simulink model "swcBrakePedalSignalingApp"  (R2022b)
settings: Solver=FixedStepDiscrete  StartTime=0  StopTime=10.0  FixedStep=0.01  RelTol=1e-3
values from neighbouring files (symbols this model uses):
  C_stopLightsSpeedThresholdSafety = Simulink.Parameter    [swcBrakePedalSignalingApp_defineIntCalibs.m]    (also in swcStopLightsMgr_defineIntCalibs.m)
  usageId = Simulink.Signal    [swcStopLightsMgr_defineIntCalibs.m]
undefined symbols (not defined in the file or in its folder): Init_stopLightASILB, pattern, STEP_BrakePedalSignalingApp, STOPLIGHTS_USAGES_DRIVER_BRAKE_PEDAL, STOPLIGHTS_USAGES_ESP_REQUEST, STOPLIGHTS_USAGES_PDC_REQUEST, usageAction, valueState
libraries: Ampere_Library x12, simulink x1
settings Model: ModifiedByFormat=Smrithi Pai  Creator=Smrithi Pai  LastModifiedBy=Smrithi Pai
settings DataIOCC: SaveOutput=off  SignalLogging=off  DSMLogging=off  SaveTime=off  ReturnWorkspaceOutputs=off
settings OptimizationCC: DefaultParameterBehavior=Inlined  EnhancedBackFolding=on  PassReuseOutputArgsAs=Individual arguments  ZeroExternalMemoryAtStartup=off  ZeroInternalMemoryAtStartup=off  LifeSpan=inf  OptimizeBlockOrder=speed  DifferentSizesBufferReuse=on  OptimizationCustomize=off  EfficientTunableParamExpr=on
settings DebuggingCC: SignalInfNanChecking=error  SignalRangeChecking=error  ReadBeforeWriteMsg=EnableAllAsError  WriteAfterWriteMsg=EnableAllAsError  WriteAfterReadMsg=EnableAllAsError  AlgebraicLoopMsg=error  ArtificialAlgebraicLoopMsg=error  SaveWithDisabledLinksMsg=error  SaveWithParameterizedLinksMsg=error  BlockPriorityViolationMsg=error  MinStepSizeMsg=error  TimeAdjustmentMsg=warning  SolverPrmCheckMsg=error  MultiTaskRateTransMsg=warning  SingleTaskRateTransMsg=warning  TasksWithSamePriorityMsg=error  SigSpecEnsureSampleTimeMsg=error  CheckMatrixSingularityMsg=error  IntegerOverflowMsg=error  ParameterUnderflowMsg=error  ParameterPrecisionLossMsg=error  ParameterTunabilityLossMsg=error  FixptConstUnderflowMsg=warning  FixptConstOverflowMsg=warning  FixptConstPrecisionLossMsg=warning  UnderSpecifiedDataTypeMsg=error  UnnecessaryDatatypeConvMsg=warning  VectorMatrixConversionMsg=error  UnconnectedInputMsg=error  UnconnectedOutputMsg=error  UnconnectedLineMsg=error  FrameProcessingCompatibilityMsg=warning  UniqueDataStoreMsg=error  BusObjectLabelMismatch=error  RootOutportRequireBusObject=error  AssertControl=DisableAll  ModelReferenceIOMsg=error  UnknownTsInhSupMsg=error  ModelReferenceDataLoggingMessage=error  StateNameClashWarn=warning  StrictBusMsg=ErrorOnBusTreatedAsVector  NonBusSignalsTreatedAsBus=error  SFUnusedDataAndEventsDiag=error  SFInvalidInputDataAccessInChartInitDiag=error  SFTransitionOutsideNaturalParentDiag=error  SFUnreachableExecutionPathDiag=error  SFUndirectedBroadcastEventsDiag=error  SFTransitionActionBeforeConditionDiag=error  SFTemporalDelaySmallerThanSampleTimeDiag=error  SFSelfTransitionDiag=error  UnderSpecifiedDimensionMsg=error  VariantConditionMismatch=error
settings ModelReferenceCC: EnableRefExpFcnMdlSchedulingChecks=on  ModelReferenceNumInstancesAllowed=Single
settings SFSimCC: SimIntegrity=alwaysOn  CompileTimeRecursionLimit=0  EnableRuntimeRecursion=off  MATLABDynamicMemAlloc=off
settings RTWCC: Description=AUTOSAR  SystemTargetFile=autosar.tlc  GenCodeOnly=on  TemplateMakefile=ert_default_tmf
settings CodeAppCC: ForceParamTrailComments=on  IgnoreCustomStorageClasses=off  OperatorAnnotations=on  SimulinkDataObjDesc=on  SFDataObjDesc=on  InsertBlockDesc=on
settings STFCustomTargetCC: TargetLangStandard=C99 (ISO)  MultiwordLength=256  ParMdlRefBuildCompliant=on  CompOptLevelCompliant=on  IncludeMdlTerminateFcn=off  CombineOutputUpdateFcns=on  SuppressErrorStatus=on  ERTCustomFileBanners=on  SupportNonFinite=off  SupportComplex=off  SupportContinuousTime=off  SupportNonInlinedSFcns=off  RemoveResetFunc=on  MATLABClassNameForMDSCustomization=Simulink.SoftwareTarget.ERTCustomization  AutosarCompliant=on  UseToolchainInfoCompliant=on  LookupTableObjectStructAxisOrder=2,1,3,4,...  LUTObjectStructOrderEvenSpacing=Size,Table,Breakpoints  SystemTargetFile=autosar.tlc
settings ERTTargetCC: TargetLangStandard=C99 (ISO)  ConcurrentExecutionCompliant=off  IncludeMdlTerminateFcn=off  SuppressErrorStatus=on  SupportNonFinite=off  SupportComplex=off  ModelStepFunctionPrototypeControlCompliant=off  CPPClassGenCompliant=off  AutosarCompliant=on  LookupTableObjectStructAxisOrder=2,1,3,4,...  LUTObjectStructOrderEvenSpacing=Size,Table,Breakpoints  InlinedParameterPlacement=NonHierarchical  ERTCustomFileTemplate=example_file_process.tlc

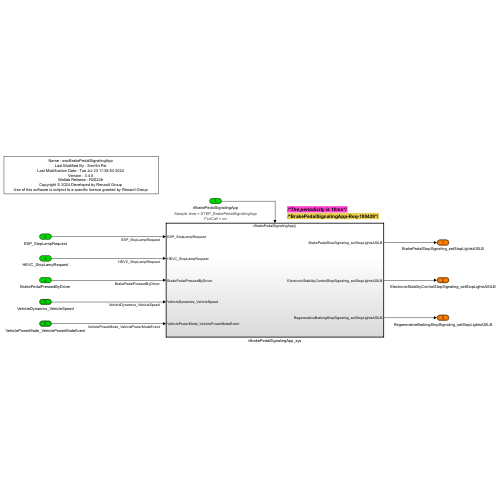
[thumbnail: Simulink's stored preview of the top-level diagram]
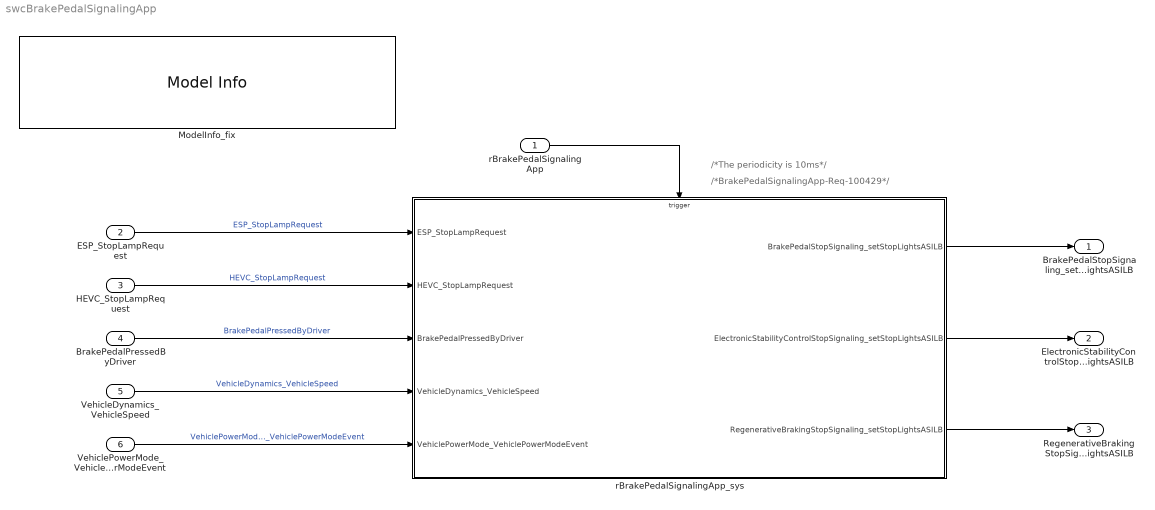
== system swcBrakePedalSignalingApp ==
  note: /*BrakePedalSignalingApp-Req-100429*/
  note: /*The periodicity is 10ms*/
  rBrakePedalSignalingApp : Inport  SampleTime=STEP_BrakePedalSignalingApp  OutputFunctionCall=on
      settings: AttributesFormatString=Sample time = %<SampleTime>\nFcnCall = %<OutputFunctionCall>
  ESP_StopLampRequest : Inport  Port=2  OutDataTypeStr=Enum: CANESPStopLampRequest  PortDimensions=1
  HEVC_StopLampRequest : Inport  Port=3  OutDataTypeStr=Enum: CANHEVCStopLampRequest  PortDimensions=1
  BrakePedalPressedByDriver : Inport  Port=4  OutDataTypeStr=Enum: CANBrakePedalPressedByDriver  PortDimensions=1  BusOutputAsStruct=on
  VehicleDynamics_VehicleSpeed : Inport  Port=5  OutDataTypeStr=Bus: VehicleSpeed  PortDimensions=1  BusOutputAsStruct=on
  VehiclePowerMode_VehiclePowerModeEvent : Inport  Port=6  OutDataTypeStr=Bus: VehiclePowerModeEvent  PortDimensions=1  BusOutputAsStruct=on
  ModelInfo_fix : simulink/Model-Wide Utilities/Model Info  Frame=on  DisplayStringWithTags=|  HorizontalTextAlignment=Center  LeftAlignmentValue=0.5
      | Name : %<ModelName>
      | Last Modified By : %<LastModifiedBy>
      | Last Modification Date : %<LastModificationDate>
      | Version : %<ModelVersion>
      | Matlab Release : R2022b
      | Copyright © 2024 Developed by Renault Group
      | Use of this software is subject to a specific licence granted by Renault Group
  rBrakePedalSignalingApp_sys : Subsystem  Description=BrakePedalSignalingApp_Req_100429
  BrakePedalStopSignaling_setStopLightsASILB : Outport  OutDataTypeStr=Bus: setStopLightsASILB  PortDimensions=1  BusOutputAsStruct=on
  ElectronicStabilityControlStopSignaling_setStopLightsASILB : Outport  Port=2  OutDataTypeStr=Bus: setStopLightsASILB  PortDimensions=1  BusOutputAsStruct=on
  RegenerativeBrakingStopSignaling_setStopLightsASILB : Outport  Port=3  OutDataTypeStr=Bus: setStopLightsASILB  PortDimensions=1  BusOutputAsStruct=on
  wires:
  rBrakePedalSignalingApp_sys/2(ElectronicStabilityControlStopSignaling_setStopLightsASILB) -> ElectronicStabilityControlStopSignaling_setStopLightsASILB/1
  rBrakePedalSignalingApp_sys/3(RegenerativeBrakingStopSignaling_setStopLightsASILB) -> RegenerativeBrakingStopSignaling_setStopLightsASILB/1
  rBrakePedalSignalingApp_sys/1(BrakePedalStopSignaling_setStopLightsASILB) -> BrakePedalStopSignaling_setStopLightsASILB/1
  VehiclePowerMode_VehiclePowerModeEvent/1 -> rBrakePedalSignalingApp_sys/5(VehiclePowerMode_VehiclePowerModeEvent)  "VehiclePowerMode_VehiclePowerModeEvent"
  VehicleDynamics_VehicleSpeed/1 -> rBrakePedalSignalingApp_sys/4(VehicleDynamics_VehicleSpeed)  "VehicleDynamics_VehicleSpeed"
  BrakePedalPressedByDriver/1 -> rBrakePedalSignalingApp_sys/3(BrakePedalPressedByDriver)  "BrakePedalPressedByDriver"
  HEVC_StopLampRequest/1 -> rBrakePedalSignalingApp_sys/2(HEVC_StopLampRequest)  "HEVC_StopLampRequest"
  ESP_StopLampRequest/1 -> rBrakePedalSignalingApp_sys/1(ESP_StopLampRequest)  "ESP_StopLampRequest"
  rBrakePedalSignalingApp/1 -> rBrakePedalSignalingApp_sys/Trigger

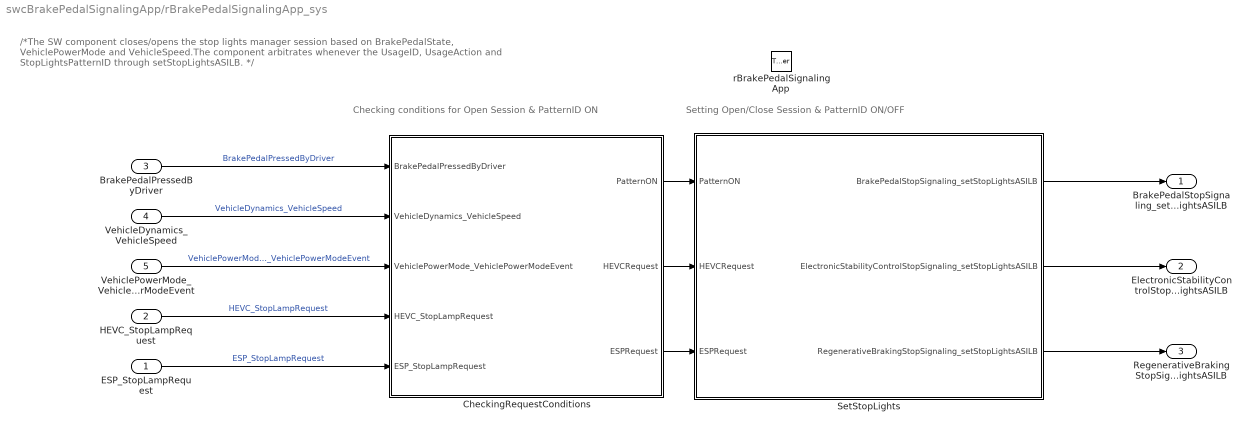
== system swcBrakePedalSignalingApp/rBrakePedalSignalingApp_sys ==
  note: Setting Open/Close Session & PatternID ON/OFF
  note: Checking conditions for Open Session & PatternID ON
  note: /*The SW component closes/opens the stop lights manager session based on BrakePedalState, VehiclePowerMode and VehicleSpeed.The component arbitrates whenever the UsageID, UsageAction and StopLightsPatternID through setStopLightsASILB. */
  ESP_StopLampRequest : Inport
  HEVC_StopLampRequest : Inport  Port=2
  BrakePedalPressedByDriver : Inport  Port=3
  VehicleDynamics_VehicleSpeed : Inport  Port=4
  VehiclePowerMode_VehiclePowerModeEvent : Inport  Port=5
  rBrakePedalSignalingApp : TriggerPort  TriggerType=function-call  VariantControl=(inherit)  SampleTimeType=periodic  SampleTime=-1
      settings: AttributesFormatString=%<StatesWhenEnabling>\n
  CheckingRequestConditions : Subsystem  TreatAsAtomicUnit=on
  SetStopLights : Subsystem  TreatAsAtomicUnit=on
  BrakePedalStopSignaling_setStopLightsASILB : Outport  InitialOutput=Init_stopLightASILB
      settings: AttributesFormatString=Init = %<InitialOutput>\n
  ElectronicStabilityControlStopSignaling_setStopLightsASILB : Outport  Port=2  InitialOutput=Init_stopLightASILB
      settings: AttributesFormatString=Init = %<InitialOutput>\n
  RegenerativeBrakingStopSignaling_setStopLightsASILB : Outport  Port=3  InitialOutput=Init_stopLightASILB
      settings: AttributesFormatString=Init = %<InitialOutput>\n
  wires:
  BrakePedalPressedByDriver/1 -> CheckingRequestConditions/1(BrakePedalPressedByDriver)  "BrakePedalPressedByDriver"
  VehicleDynamics_VehicleSpeed/1 -> CheckingRequestConditions/2(VehicleDynamics_VehicleSpeed)  "VehicleDynamics_VehicleSpeed"
  VehiclePowerMode_VehiclePowerModeEvent/1 -> CheckingRequestConditions/3(VehiclePowerMode_VehiclePowerModeEvent)  "VehiclePowerMode_VehiclePowerModeEvent"
  CheckingRequestConditions/1(PatternON) -> SetStopLights/1(PatternON)
  SetStopLights/1(BrakePedalStopSignaling_setStopLightsASILB) -> BrakePedalStopSignaling_setStopLightsASILB/1
  HEVC_StopLampRequest/1 -> CheckingRequestConditions/4(HEVC_StopLampRequest)  "HEVC_StopLampRequest"
  ESP_StopLampRequest/1 -> CheckingRequestConditions/5(ESP_StopLampRequest)  "ESP_StopLampRequest"
  CheckingRequestConditions/2(HEVCRequest) -> SetStopLights/2(HEVCRequest)
  CheckingRequestConditions/3(ESPRequest) -> SetStopLights/3(ESPRequest)
  SetStopLights/2(ElectronicStabilityControlStopSignaling_setStopLightsASILB) -> ElectronicStabilityControlStopSignaling_setStopLightsASILB/1
  SetStopLights/3(RegenerativeBrakingStopSignaling_setStopLightsASILB) -> RegenerativeBrakingStopSignaling_setStopLightsASILB/1

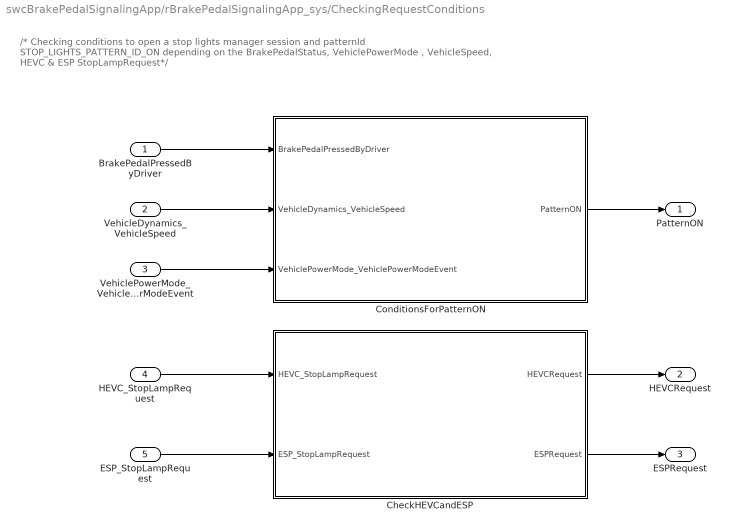
== system swcBrakePedalSignalingApp/rBrakePedalSignalingApp_sys/CheckingRequestConditions ==
  note: /* Checking conditions to open a stop lights manager session and patternId STOP_LIGHTS_PATTERN_ID_ON depending on the BrakePedalStatus, VehiclePowerMode , VehicleSpeed, HEVC & ESP StopLampRequest*/
  BrakePedalPressedByDriver : Inport
  VehicleDynamics_VehicleSpeed : Inport  Port=2
  VehiclePowerMode_VehiclePowerModeEvent : Inport  Port=3
  HEVC_StopLampRequest : Inport  Port=4
  ESP_StopLampRequest : Inport  Port=5
  CheckHEVCandESP : Subsystem  Description=|  TreatAsAtomicUnit=on
      | ESPSignalingApp_Req_100425
      | HEVCSignalingApp_Req_100427
  ConditionsForPatternON : Subsystem  Description=|  TreatAsAtomicUnit=on
      | BrakePedalSignalingApp_Req_100430
      | BrakePedalSignalingApp_Req_100431
  PatternON : Outport
  HEVCRequest : Outport  Port=2
  ESPRequest : Outport  Port=3
  wires:
  BrakePedalPressedByDriver/1 -> ConditionsForPatternON/1(BrakePedalPressedByDriver)
  VehicleDynamics_VehicleSpeed/1 -> ConditionsForPatternON/2(VehicleDynamics_VehicleSpeed)
  VehiclePowerMode_VehiclePowerModeEvent/1 -> ConditionsForPatternON/3(VehiclePowerMode_VehiclePowerModeEvent)
  HEVC_StopLampRequest/1 -> CheckHEVCandESP/1(HEVC_StopLampRequest)
  ESP_StopLampRequest/1 -> CheckHEVCandESP/2(ESP_StopLampRequest)
  ConditionsForPatternON/1(PatternON) -> PatternON/1
  CheckHEVCandESP/1(HEVCRequest) -> HEVCRequest/1
  CheckHEVCandESP/2(ESPRequest) -> ESPRequest/1

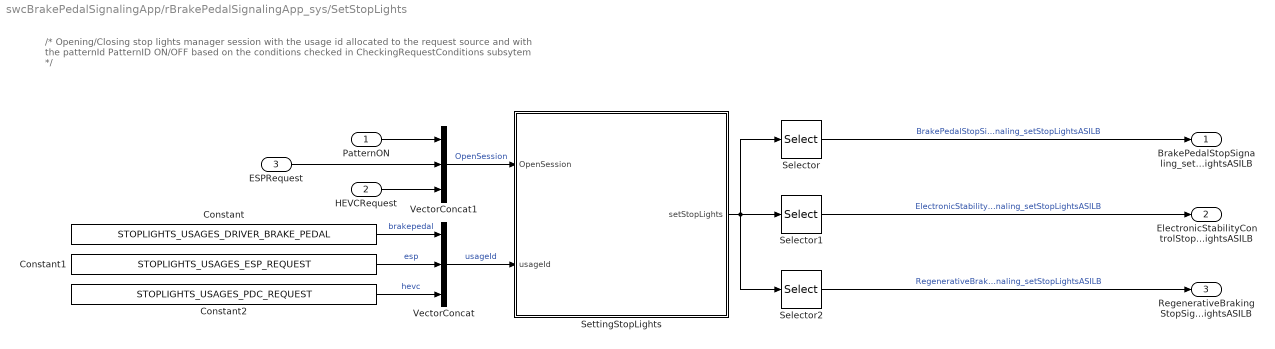
== system swcBrakePedalSignalingApp/rBrakePedalSignalingApp_sys/SetStopLights ==
  note: /* Opening/Closing stop lights manager session with the usage id allocated to the request source and with the patternId PatternID ON/OFF based on the conditions checked in CheckingRequestConditions subsytem */
  PatternON : Inport
  HEVCRequest : Inport  Port=2
  ESPRequest : Inport  Port=3
  Constant : Constant  Value=STOPLIGHTS_USAGES_DRIVER_BRAKE_PEDAL
  Constant1 : Constant  Value=STOPLIGHTS_USAGES_ESP_REQUEST
  Constant2 : Constant  Value=STOPLIGHTS_USAGES_PDC_REQUEST
  Selector : Selector  InputPortWidth=3  IndexOptions=Index vector (dialog)  Indices=[1]  OutputSizes=1
      settings: AttributesFormatString=%<IndexMode>\n
  Selector1 : Selector  InputPortWidth=3  IndexOptions=Index vector (dialog)  Indices=[2]  OutputSizes=1
      settings: AttributesFormatString=%<IndexMode>\n
  Selector2 : Selector  InputPortWidth=3  IndexOptions=Index vector (dialog)  Indices=[3]  OutputSizes=1
      settings: AttributesFormatString=%<IndexMode>\n
  SettingStopLights : Subsystem  Description=|  TreatAsAtomicUnit=on
      | BrakePedalSignalingApp_Req_100403
      | ESPSignalingApp_Req_100425
      | ESPSignalingApp_Req_100426
      | HEVCSignalingApp_Req_100427
      | HEVCSignalingApp_Req_100428
      | BrakePedalSignalingApp_Req_100430
      | BrakePedalSignalingApp_Req_100431
      | BrakePedalSignalingApp_Req_100432
      | BrakePedalSignalingApp_Req_100433
  VectorConcat : Concatenate  NumInputs=3
  VectorConcat1 : Concatenate  NumInputs=3
  BrakePedalStopSignaling_setStopLightsASILB : Outport
  ElectronicStabilityControlStopSignaling_setStopLightsASILB : Outport  Port=2
  RegenerativeBrakingStopSignaling_setStopLightsASILB : Outport  Port=3
  wires:
  SettingStopLights/1(setStopLights) -> Selector1/1, Selector/1, Selector2/1
  Selector/1 -> BrakePedalStopSignaling_setStopLightsASILB/1  "BrakePedalStopSignaling_setStopLightsASILB"
  Selector1/1 -> ElectronicStabilityControlStopSignaling_setStopLightsASILB/1  "ElectronicStabilityControlStopSignaling_setStopLightsASILB"
  Selector2/1 -> RegenerativeBrakingStopSignaling_setStopLightsASILB/1  "RegenerativeBrakingStopSignaling_setStopLightsASILB"
  Constant/1 -> VectorConcat/1  "brakepedal"
  Constant1/1 -> VectorConcat/2  "esp"
  Constant2/1 -> VectorConcat/3  "hevc"
  VectorConcat/1 -> SettingStopLights/2(usageId)  "usageId"
  VectorConcat1/1 -> SettingStopLights/1(OpenSession)  "OpenSession"
  PatternON/1 -> VectorConcat1/1
  HEVCRequest/1 -> VectorConcat1/3
  ESPRequest/1 -> VectorConcat1/2

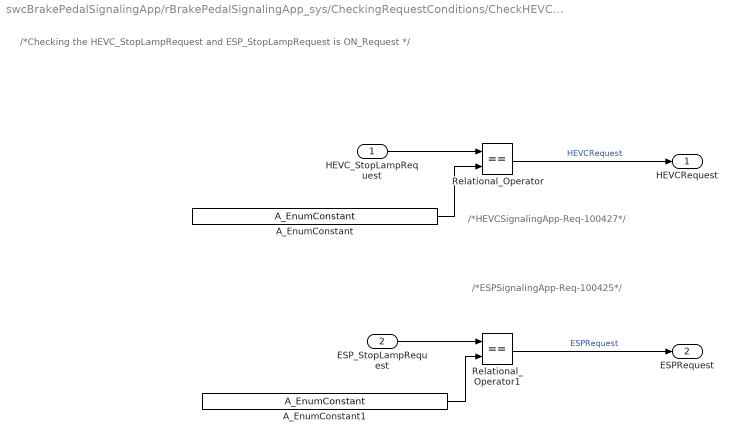
== system swcBrakePedalSignalingApp/rBrakePedalSignalingApp_sys/CheckingRequestConditions/CheckHEVCandESP ==
  note: /*ESPSignalingApp-Req-100425*/
  note: /*Checking the HEVC_StopLampRequest and ESP_StopLampRequest is ON_Request */
  note: /*HEVCSignalingApp-Req-100427*/
  HEVC_StopLampRequest : Inport
  ESP_StopLampRequest : Inport  Port=2
  A_EnumConstant : Ampere_Library/User_Defined_Libraries/Sources/A_EnumConstant  Tag=[LIB]  OutDataTypeStr=Enum: CANHEVCStopLampRequest  EnumVal=CANHEVCSTOPLAMPREQUEST_ON_REQUEST
      settings: AttributesFormatString=Enum: CANHEVCStopLampRequest
  A_EnumConstant1 : Ampere_Library/User_Defined_Libraries/Sources/A_EnumConstant  Tag=[LIB]  OutDataTypeStr=Enum: CANESPStopLampRequest  EnumVal=CANESPSTOPLAMPREQUEST_ON_REQUESTED
      settings: AttributesFormatString=Enum: CANESPStopLampRequest
  Relational_Operator : RelationalOperator  Operator===  OutDataTypeStr=boolean  RndMeth=Zero
  Relational_Operator1 : RelationalOperator  Operator===  OutDataTypeStr=boolean  RndMeth=Zero
  HEVCRequest : Outport
  ESPRequest : Outport  Port=2
  wires:
  A_EnumConstant/1 -> Relational_Operator/2
  HEVC_StopLampRequest/1 -> Relational_Operator/1
  Relational_Operator/1 -> HEVCRequest/1  "HEVCRequest"
  A_EnumConstant1/1 -> Relational_Operator1/2
  ESP_StopLampRequest/1 -> Relational_Operator1/1
  Relational_Operator1/1 -> ESPRequest/1  "ESPRequest"

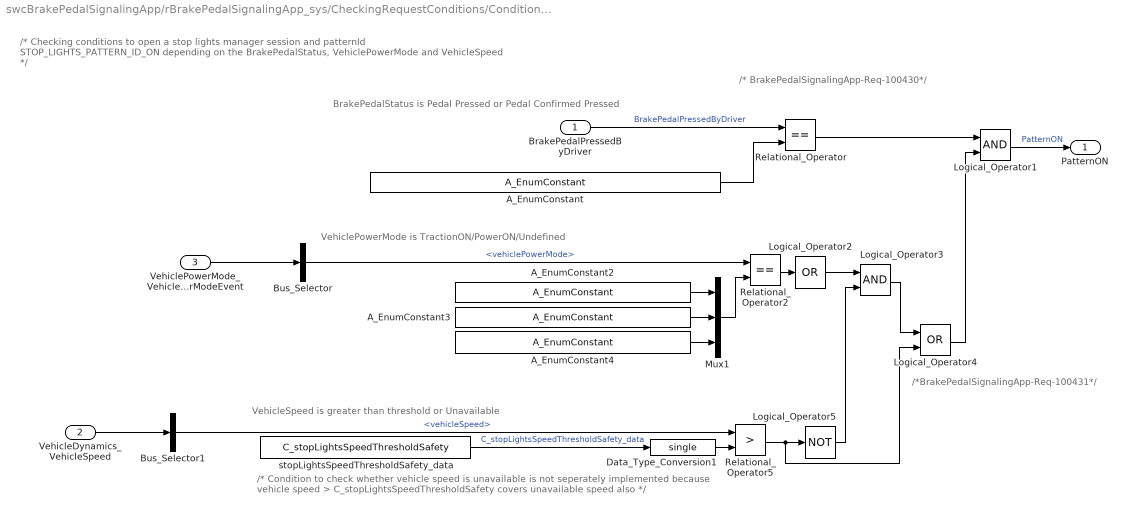
== system swcBrakePedalSignalingApp/rBrakePedalSignalingApp_sys/CheckingRequestConditions/ConditionsForPatternON ==
  note: /* Checking conditions to open a stop lights manager session and patternId STOP_LIGHTS_PATTERN_ID_ON depending on the BrakePedalStatus, VehiclePowerMode and VehicleSpeed */
  note: VehiclePowerMode is TractionON/PowerON/Undefined
  note: /*BrakePedalSignalingApp-Req-100431*/
  note: /* BrakePedalSignalingApp-Req-100430*/
  note: VehicleSpeed is greater than threshold or Unavailable
  note: BrakePedalStatus is Pedal Pressed or Pedal Confirmed Pressed
  note: /* Condition to check whether vehicle speed is unavailable is not seperately implemented because vehicle speed > C_stopLightsSpeedThresholdSafety covers unavailable speed also */
  BrakePedalPressedByDriver : Inport
  VehicleDynamics_VehicleSpeed : Inport  Port=2
  VehiclePowerMode_VehiclePowerModeEvent : Inport  Port=3
  A_EnumConstant : Ampere_Library/User_Defined_Libraries/Sources/A_EnumConstant  Tag=[LIB]  OutDataTypeStr=Enum: CANBrakePedalPressedByDriver  EnumVal=CANBRAKEPEDALPRESSEDBYDRIVER_PRESSED
      settings: AttributesFormatString=Enum: CANBrakePedalPressedByDriver
  A_EnumConstant2 : Ampere_Library/User_Defined_Libraries/Sources/A_EnumConstant  Tag=[LIB]  OutDataTypeStr=Enum: VehiclePowerModeType  EnumVal=VEHICLEPOWERMODE_TRACTION_ON
      settings: AttributesFormatString=Enum: VehiclePowerModeType
  A_EnumConstant3 : Ampere_Library/User_Defined_Libraries/Sources/A_EnumConstant  Tag=[LIB]  OutDataTypeStr=Enum: VehiclePowerModeType  EnumVal=VEHICLEPOWERMODE_POWER_ON
      settings: AttributesFormatString=Enum: VehiclePowerModeType
  A_EnumConstant4 : Ampere_Library/User_Defined_Libraries/Sources/A_EnumConstant  Tag=[LIB]  OutDataTypeStr=Enum: VehiclePowerModeType  EnumVal=VEHICLEPOWERMODE_UNDEFINED
      settings: AttributesFormatString=Enum: VehiclePowerModeType
  Bus_Selector : BusSelector  OutputSignals=vehiclePowerMode
  Bus_Selector1 : BusSelector  OutputSignals=vehicleSpeed
  Data_Type_Conversion1 : DataTypeConversion  OutDataTypeStr=single  SaturateOnIntegerOverflow=off
  Logical_Operator1 : Logic  OutDataTypeStr=boolean
  Logical_Operator2 : Logic  Operator=OR  Inputs=1  OutDataTypeStr=boolean
  Logical_Operator3 : Logic  OutDataTypeStr=boolean
  Logical_Operator4 : Logic  Operator=OR  OutDataTypeStr=boolean
  Logical_Operator5 : Logic  Operator=NOT  Inputs=1  OutDataTypeStr=boolean
  Mux1 : Mux  Inputs=3
  Relational_Operator : RelationalOperator  Operator===  OutDataTypeStr=boolean  RndMeth=Zero
  Relational_Operator2 : RelationalOperator  Operator===  OutDataTypeStr=boolean  RndMeth=Zero
  Relational_Operator5 : RelationalOperator  Operator=>  OutDataTypeStr=boolean  RndMeth=Zero
  stopLightsSpeedThresholdSafety_data : Constant  Value=C_stopLightsSpeedThresholdSafety
  PatternON : Outport
  wires:
  Bus_Selector1/1 -> Relational_Operator5/1  "<vehicleSpeed>"
  A_EnumConstant3/1 -> Mux1/2
  Relational_Operator5/1 -> Logical_Operator4/2, Logical_Operator5/1
  Logical_Operator5/1 -> Logical_Operator3/2
  Relational_Operator/1 -> Logical_Operator1/1
  Mux1/1 -> Relational_Operator2/2
  Logical_Operator3/1 -> Logical_Operator4/1
  A_EnumConstant2/1 -> Mux1/1
  BrakePedalPressedByDriver/1 -> Relational_Operator/1  "BrakePedalPressedByDriver"
  Logical_Operator1/1 -> PatternON/1  "PatternON"
  VehiclePowerMode_VehiclePowerModeEvent/1 -> Bus_Selector/1
  A_EnumConstant4/1 -> Mux1/3
  Data_Type_Conversion1/1 -> Relational_Operator5/2
  stopLightsSpeedThresholdSafety_data/1 -> Data_Type_Conversion1/1  "C_stopLightsSpeedThresholdSafety_data"
  Logical_Operator2/1 -> Logical_Operator3/1
  VehicleDynamics_VehicleSpeed/1 -> Bus_Selector1/1
  Relational_Operator2/1 -> Logical_Operator2/1
  Bus_Selector/1 -> Relational_Operator2/1  "<vehiclePowerMode>"
  Logical_Operator4/1 -> Logical_Operator1/2
  A_EnumConstant/1 -> Relational_Operator/2

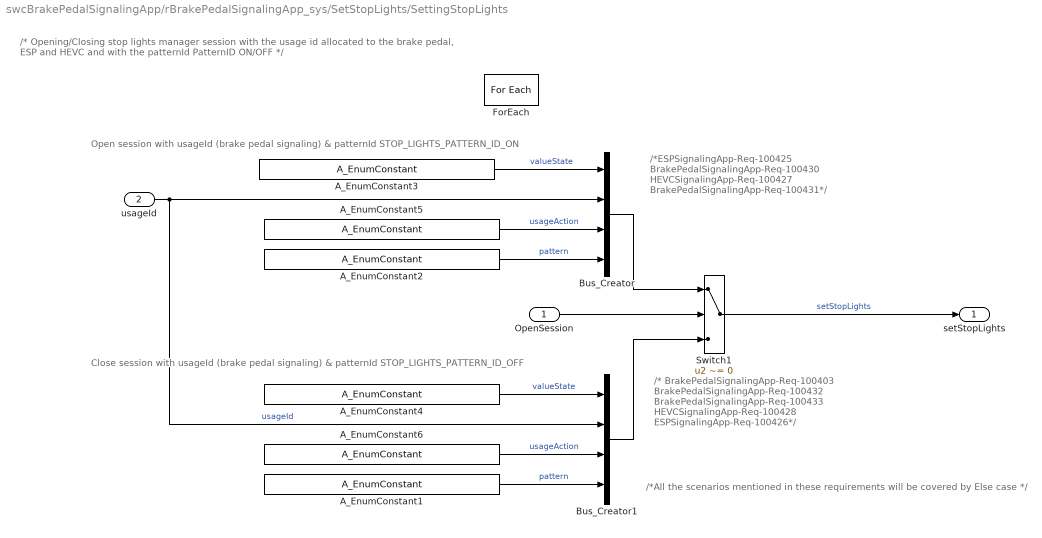
== system swcBrakePedalSignalingApp/rBrakePedalSignalingApp_sys/SetStopLights/SettingStopLights ==
  note: /*ESPSignalingApp-Req-100425
      | BrakePedalSignalingApp-Req-100430
      | HEVCSignalingApp-Req-100427
      | BrakePedalSignalingApp-Req-100431*/
  note: /* Opening/Closing stop lights manager session with the usage id allocated to the brake pedal, ESP and HEVC and with the patternId PatternID ON/OFF */
  note: Open session with usageId (brake pedal signaling) & patternId STOP_LIGHTS_PATTERN_ID_ON
  note: Close session with usageId (brake pedal signaling) & patternId STOP_LIGHTS_PATTERN_ID_OFF
  note: /*All the scenarios mentioned in these requirements will be covered by Else case */
  note: /* BrakePedalSignalingApp-Req-100403
      | BrakePedalSignalingApp-Req-100432
      | BrakePedalSignalingApp-Req-100433
      | HEVCSignalingApp-Req-100428
      | ESPSignalingApp-Req-100426*/
  OpenSession : Inport  Partition=on  PartitionDimension=1  PartitionWidth=1  PartitionOffset=0
  usageId : Inport  Port=2  Partition=on  PartitionDimension=1  PartitionWidth=1  PartitionOffset=0
  A_EnumConstant1 : Ampere_Library/User_Defined_Libraries/Sources/A_EnumConstant  Tag=[LIB]  OutDataTypeStr=Enum: StopLightsPatternID  EnumVal=STOP_LIGHTS_PATTERN_ID_OFF
      settings: AttributesFormatString=Enum: StopLightsPatternID
  A_EnumConstant2 : Ampere_Library/User_Defined_Libraries/Sources/A_EnumConstant  Tag=[LIB]  OutDataTypeStr=Enum: StopLightsPatternID  EnumVal=STOP_LIGHTS_PATTERN_ID_ON
      settings: AttributesFormatString=Enum: StopLightsPatternID
  A_EnumConstant3 : Ampere_Library/User_Defined_Libraries/Sources/A_EnumConstant  Tag=[LIB]  OutDataTypeStr=Enum: ValueState  EnumVal=VALUE_STATE_VALID
      settings: AttributesFormatString=Enum: ValueState
  A_EnumConstant4 : Ampere_Library/User_Defined_Libraries/Sources/A_EnumConstant  Tag=[LIB]  OutDataTypeStr=Enum: ValueState  EnumVal=VALUE_STATE_VALID
      settings: AttributesFormatString=Enum: ValueState
  A_EnumConstant5 : Ampere_Library/User_Defined_Libraries/Sources/A_EnumConstant  Tag=[LIB]  OutDataTypeStr=Enum: UsageAction  EnumVal=USAGEACTION_OPEN_SESSION
      settings: AttributesFormatString=Enum: UsageAction
  A_EnumConstant6 : Ampere_Library/User_Defined_Libraries/Sources/A_EnumConstant  Tag=[LIB]  OutDataTypeStr=Enum: UsageAction  EnumVal=USAGEACTION_CLOSE_SESSION
      settings: AttributesFormatString=Enum: UsageAction
  Bus_Creator : BusCreator  Inputs=valueState,usageId,usageAction,pattern  OutDataTypeStr=Bus: setStopLightsASILB  NonVirtualBus=on
  Bus_Creator1 : BusCreator  Inputs=valueState,usageId,usageAction,pattern  OutDataTypeStr=Bus: setStopLightsASILB  NonVirtualBus=on
  ForEach : ForEach  DisableCoverage=on
  Switch1 : Switch  Criteria=u2 ~= 0  RndMeth=Zero  SaturateOnIntegerOverflow=off
  setStopLights : Outport  ConcatenationDimension=1
  wires:
  A_EnumConstant6/1 -> Bus_Creator1/3  "usageAction"
  A_EnumConstant1/1 -> Bus_Creator1/4  "pattern"
  Bus_Creator1/1 -> Switch1/3
  A_EnumConstant5/1 -> Bus_Creator/3  "usageAction"
  A_EnumConstant3/1 -> Bus_Creator/1  "valueState"
  OpenSession/1 -> Switch1/2
  Bus_Creator/1 -> Switch1/1
  A_EnumConstant4/1 -> Bus_Creator1/1  "valueState"
  usageId/1 -> Bus_Creator/2, Bus_Creator1/2  "usageId"
  A_EnumConstant2/1 -> Bus_Creator/4  "pattern"
  Switch1/1 -> setStopLights/1  "setStopLights"
